simulink model "Controller"  (R2018b)
settings: configuration reference "control_config" (kept outside this file)
values from neighbouring files (symbols this model uses):
  CONTROL_EXPORT = Simulink.Parameter(CONTROL_EXPORT_VALUE)    [controller_model_init.m]
  CONTROL_PARAM = Simulink.Parameter(CONTROL_PARAM_VALUE)    [controller_model_init.m]
undefined symbols (not defined in the file or in its folder): actuator_cmd, ControlMode, DiscIntNeverNeededParam, timestamp
libraries: FMT_Model_Lib x2, simulink x1
settings Model: Creator=jc  LastModifiedBy=zouji
settings ConfigSetRef: SourceLocation=Base Workspace

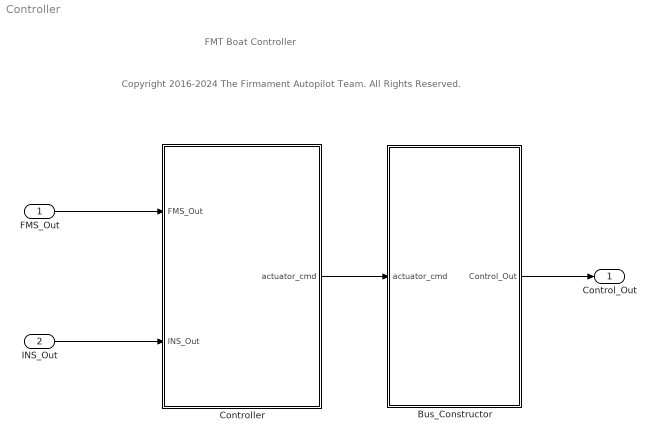
== system Controller ==
  note: FMT Boat Controller
  note: Copyright 2016-2024 The Firmament Autopilot Team. All Rights Reserved.
  FMS_Out : Inport  OutDataTypeStr=Bus: FMS_Out_Bus
  INS_Out : Inport  Port=2  OutDataTypeStr=Bus: INS_Out_Bus
  Bus_Constructor : Subsystem
  Controller : Subsystem
  Control_Out : Outport  OutDataTypeStr=Bus: Control_Out_Bus
  wires:
  Bus_Constructor/1(Control_Out) -> Control_Out/1
  INS_Out/1 -> Controller/2(INS_Out)
  FMS_Out/1 -> Controller/1(FMS_Out)
  Controller/1(actuator_cmd) -> Bus_Constructor/1(actuator_cmd)

== system Controller/Bus_Constructor ==
  actuator_cmd : Inport
  Bus Assignment : BusAssignment  AssignedSignals=actuator_cmd,timestamp
  Constant : Constant  Value=0  OutDataTypeStr=Bus: Control_Out_Bus
  timestamp : Subsystem  mask{sample_time=CONTROL_EXPORT.period}
      mask prompts: sample_time "sample time (ms)"
  Control_Out : Outport
  wires:
  actuator_cmd/1 -> Bus Assignment/2
  Constant/1 -> Bus Assignment/1
  Bus Assignment/1 -> Control_Out/1
  timestamp/1(timestamp_ms) -> Bus Assignment/3

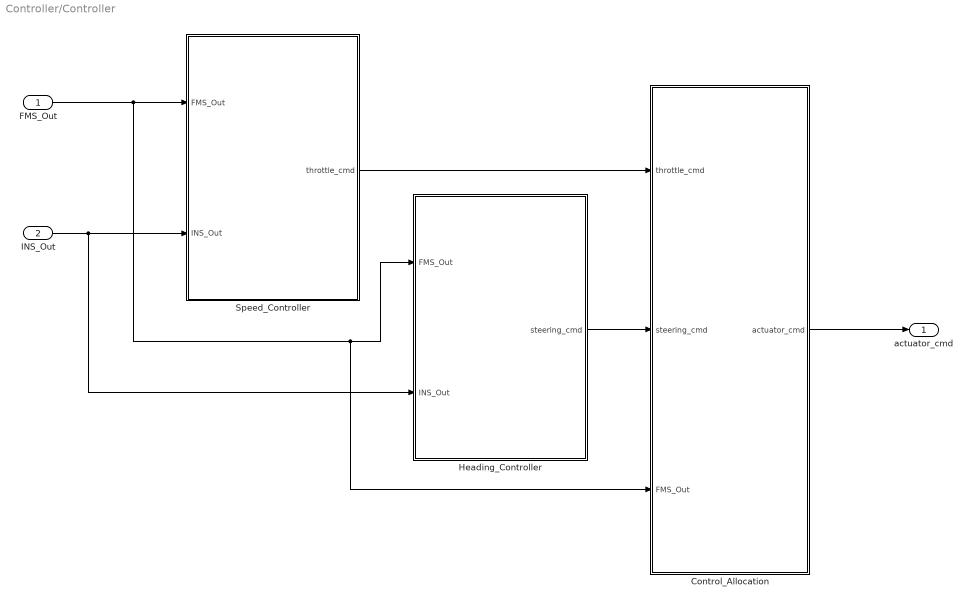
== system Controller/Controller ==
  FMS_Out : Inport
  INS_Out : Inport  Port=2
  Control_Allocation : Subsystem  Variant=on
      settings: GeneratePreprocessorConditionals=on
  Heading_Controller : Subsystem
  Speed_Controller : Subsystem
  actuator_cmd : Outport
  wires:
  FMS_Out/1 -> Control_Allocation/3(FMS_Out), Heading_Controller/1(FMS_Out), Speed_Controller/1(FMS_Out)
  INS_Out/1 -> Heading_Controller/2(INS_Out), Speed_Controller/2(INS_Out)
  Control_Allocation/1(actuator_cmd) -> actuator_cmd/1
  Speed_Controller/1(throttle_cmd) -> Control_Allocation/1(throttle_cmd)
  Heading_Controller/1(steering_cmd) -> Control_Allocation/2(steering_cmd)

== system Controller/Bus_Constructor/timestamp ==
  Constant : Constant  Value=sample_time
  Data Type Conversion : DataTypeConversion  OutDataTypeStr=uint32
  Discrete-Time Integrator : DiscreteIntegrator  IntegratorMethod=Accumulation: Forward Euler  SampleTime=-1  ICPrevOutput=DiscIntNeverNeededParam  ICPrevScaledInput=DiscIntNeverNeededParam
  timestamp_ms : Outport
  wires:
  Discrete-Time Integrator/1 -> Data Type Conversion/1
  Constant/1 -> Discrete-Time Integrator/1
  Data Type Conversion/1 -> timestamp_ms/1

== system Controller/Controller/Control_Allocation ==
  note: 1) Add Subsystem or Model blocks as valid variant choices.
      | 2) You cannot connect blocks at this level. At simulation, connectivity is automatically
      | determined, based on the active variant and port name matching.
  throttle_cmd : Inport
  steering_cmd : Inport  Port=2
  FMS_Out : Inport  Port=3
  Boat_1 : Subsystem  TreatAsAtomicUnit=on  VariantControl=AIRFRAME==1
      mask Display: image('D:\ws\FMT\FMT-Model\figures\boat_1.png');
  actuator_cmd : Outport

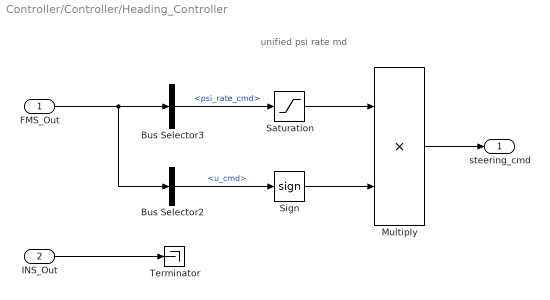
== system Controller/Controller/Heading_Controller ==
  note: unified psi rate md
  FMS_Out : Inport
  INS_Out : Inport  Port=2
  Bus Selector2 : BusSelector  OutputSignals=u_cmd
  Bus Selector3 : BusSelector  OutputSignals=psi_rate_cmd
  Multiply : Product
  Saturation : Saturate  UpperLimit=1  LowerLimit=-1
  Sign : Signum
  Terminator : Terminator
  steering_cmd : Outport
  wires:
  INS_Out/1 -> Terminator/1
  Sign/1 -> Multiply/2
  Bus Selector2/1 -> Sign/1  "<u_cmd>"
  Saturation/1 -> Multiply/1
  Multiply/1 -> steering_cmd/1
  Bus Selector3/1 -> Saturation/1  "<psi_rate_cmd>"
  FMS_Out/1 -> Bus Selector3/1, Bus Selector2/1

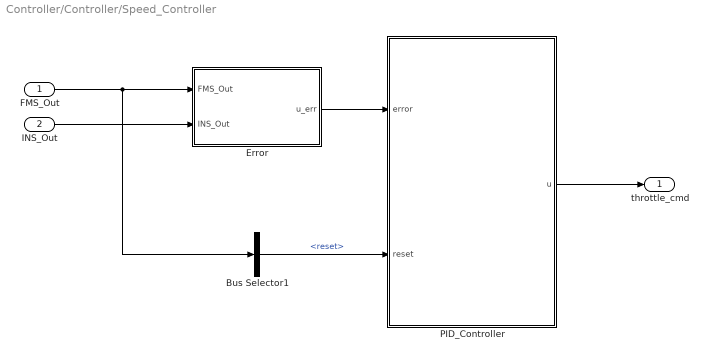
== system Controller/Controller/Speed_Controller ==
  FMS_Out : Inport
  INS_Out : Inport  Port=2
  Bus Selector1 : BusSelector  OutputSignals=reset
  Error : Subsystem
  PID_Controller : Subsystem
  throttle_cmd : Outport
  wires:
  Bus Selector1/1 -> PID_Controller/2(reset)  "<reset>"
  FMS_Out/1 -> Bus Selector1/1, Error/1(FMS_Out)
  Error/1(u_err) -> PID_Controller/1(error)
  PID_Controller/1(u) -> throttle_cmd/1
  INS_Out/1 -> Error/2(INS_Out)

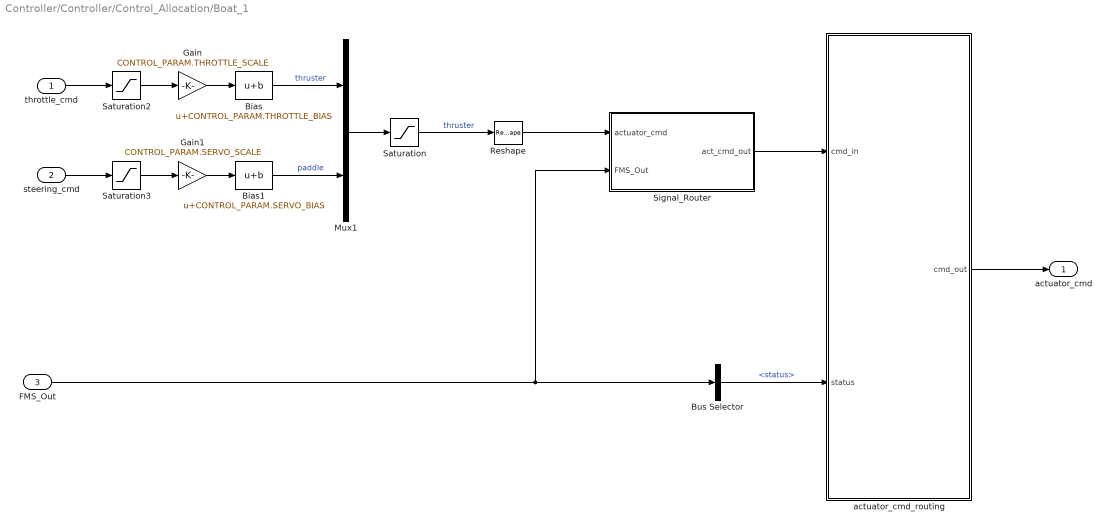
== system Controller/Controller/Control_Allocation/Boat_1 ==
  throttle_cmd : Inport
  steering_cmd : Inport  Port=2
  FMS_Out : Inport  Port=3
  Bias : Bias  Bias=CONTROL_PARAM.THROTTLE_BIAS
  Bias1 : Bias  Bias=CONTROL_PARAM.SERVO_BIAS
  Bus Selector : BusSelector  OutputSignals=status
  Gain : Gain  Gain=CONTROL_PARAM.THROTTLE_SCALE  OutDataTypeStr=uint16
  Gain1 : Gain  Gain=CONTROL_PARAM.SERVO_SCALE  OutDataTypeStr=uint16
  Mux1 : Mux  Inputs=2
  Reshape : Reshape  OutputDimensionality=Column vector (2-D)
  Saturation : Saturate  UpperLimit=2000  LowerLimit=1000
  Saturation2 : Saturate  UpperLimit=1  LowerLimit=-1
  Saturation3 : Saturate  UpperLimit=1  LowerLimit=-1
  Signal_Router : Subsystem
  actuator_cmd_routing : Subsystem
  actuator_cmd : Outport
  wires:
  Bias1/1 -> Mux1/2  "paddle"
  Gain1/1 -> Bias1/1
  Gain/1 -> Bias/1
  throttle_cmd/1 -> Saturation2/1
  steering_cmd/1 -> Saturation3/1
  Bias/1 -> Mux1/1  "thruster"
  Reshape/1 -> Signal_Router/1(actuator_cmd)
  Bus Selector/1 -> actuator_cmd_routing/2(status)  "<status>"
  Signal_Router/1(act_cmd_out) -> actuator_cmd_routing/1(cmd_in)
  FMS_Out/1 -> Signal_Router/2(FMS_Out), Bus Selector/1
  Mux1/1 -> Saturation/1
  actuator_cmd_routing/1(cmd_out) -> actuator_cmd/1
  Saturation2/1 -> Gain/1
  Saturation3/1 -> Gain1/1
  Saturation/1 -> Reshape/1  "thruster"

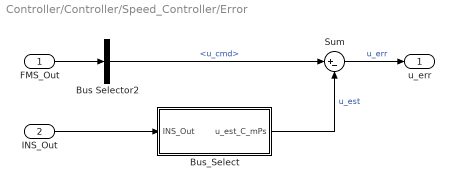
== system Controller/Controller/Speed_Controller/Error ==
  FMS_Out : Inport
  INS_Out : Inport  Port=2
  Bus Selector2 : BusSelector  OutputSignals=u_cmd
  Bus_Select : Subsystem
  Sum : Sum  Inputs=|+-
  u_err : Outport
  wires:
  FMS_Out/1 -> Bus Selector2/1
  INS_Out/1 -> Bus_Select/1(INS_Out)
  Bus_Select/1(u_est_C_mPs) -> Sum/2  "u_est"
  Bus Selector2/1 -> Sum/1  "<u_cmd>"
  Sum/1 -> u_err/1  "u_err"

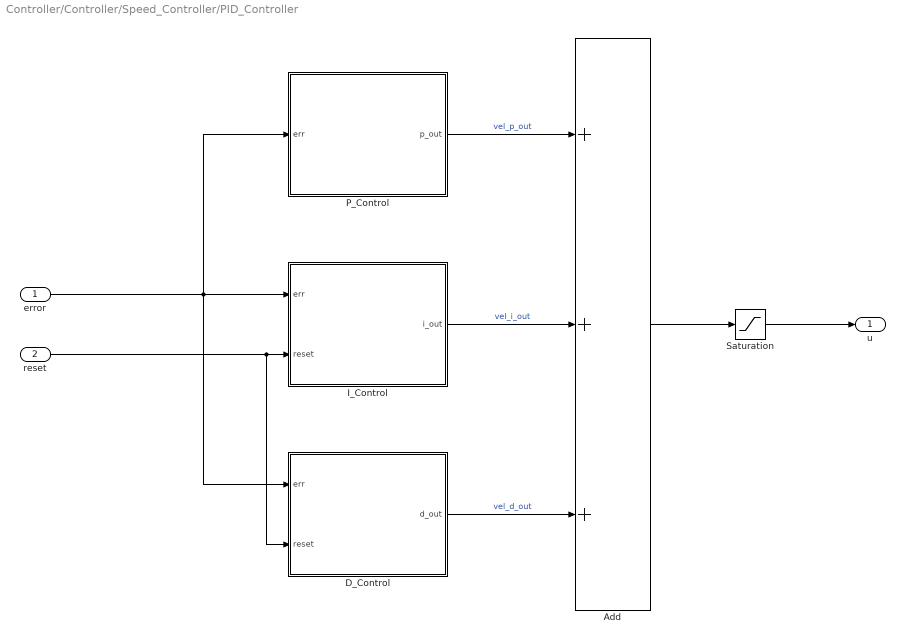
== system Controller/Controller/Speed_Controller/PID_Controller ==
  error : Inport
  reset : Inport  Port=2
  Add : Sum  Inputs=+++
  D_Control : Subsystem  mask{kd=CONTROL_PARAM.VEL_D, max_d=CONTROL_PARAM.VEL_D_MAX, min_d=CONTROL_PARAM.VEL_D_MIN}
  I_Control : Subsystem  mask{ki=CONTROL_PARAM.VEL_I, max_i=CONTROL_PARAM.VEL_I_MAX, min_i=CONTROL_PARAM.VEL_I_MIN}
  P_Control : Subsystem  mask{kp=CONTROL_PARAM.VEL_P}
  Saturation : Saturate  UpperLimit=1  LowerLimit=-1
  u : Outport
  wires:
  error/1 -> P_Control/1(err), I_Control/1(err), D_Control/1(err)
  P_Control/1(p_out) -> Add/1  "vel_p_out"
  I_Control/1(i_out) -> Add/2  "vel_i_out"
  D_Control/1(d_out) -> Add/3  "vel_d_out"
  reset/1 -> I_Control/2(reset), D_Control/2(reset)
  Add/1 -> Saturation/1
  Saturation/1 -> u/1

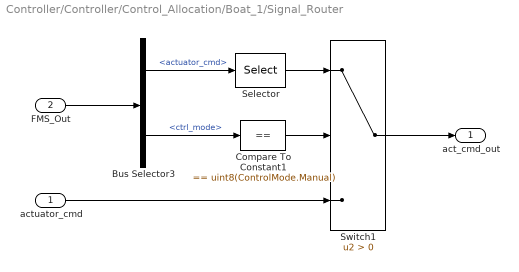
== system Controller/Controller/Control_Allocation/Boat_1/Signal_Router ==
  actuator_cmd : Inport
  FMS_Out : Inport  Port=2
  Bus Selector3 : BusSelector  OutputSignals=actuator_cmd,ctrl_mode
  Compare To Constant1 : simulink/Logic and Bit Operations/Compare To Constant  relop===  const=uint8(ControlMode.Manual)  OutDataTypeStr=boolean
  Selector : Selector  InputPortWidth=16  IndexOptions=Index vector (dialog)  Indices=[1 2]  OutputSizes=1
  Switch1 : Switch  Criteria=u2 > Threshold
  act_cmd_out : Outport
  wires:
  Compare To Constant1/1 -> Switch1/2
  Bus Selector3/1 -> Selector/1  "<actuator_cmd>"
  Bus Selector3/2 -> Compare To Constant1/1  "<ctrl_mode>"
  actuator_cmd/1 -> Switch1/3
  FMS_Out/1 -> Bus Selector3/1
  Switch1/1 -> act_cmd_out/1
  Selector/1 -> Switch1/1

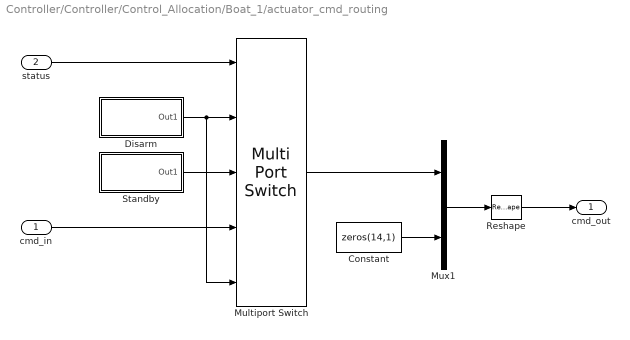
== system Controller/Controller/Control_Allocation/Boat_1/actuator_cmd_routing ==
  cmd_in : Inport
  status : Inport  Port=2
  Constant : Constant  Value=zeros(14,1)  VectorParams1D=off  OutDataTypeStr=uint16
  Disarm : Subsystem
  Multiport Switch : MultiPortSwitch  DataPortForDefault=Additional data port  DiagnosticForDefault=None
  Mux1 : Mux  Inputs=2
  Reshape : Reshape  OutputDimensionality=Customize  OutputDimensions=[16,1]
  Standby : Subsystem
  cmd_out : Outport
  wires:
  Reshape/1 -> cmd_out/1
  Constant/1 -> Mux1/2
  Mux1/1 -> Reshape/1
  status/1 -> Multiport Switch/1
  Multiport Switch/1 -> Mux1/1
  cmd_in/1 -> Multiport Switch/4
  Disarm/1(Out1) -> Multiport Switch/5, Multiport Switch/2
  Standby/1(Out1) -> Multiport Switch/3

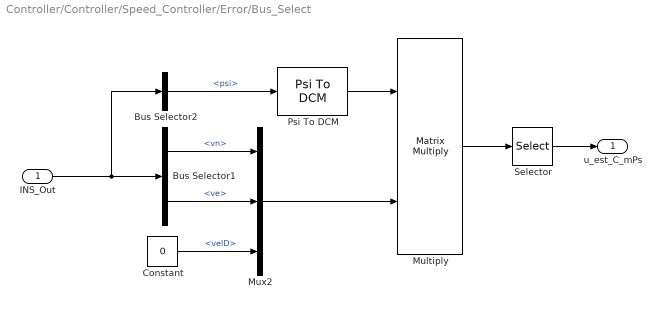
== system Controller/Controller/Speed_Controller/Error/Bus_Select ==
  INS_Out : Inport
  Bus Selector1 : BusSelector  OutputSignals=vn,ve
  Bus Selector2 : BusSelector  OutputSignals=psi
  Constant : Constant  Value=0  OutDataTypeStr=single
  Multiply : Product  Multiplication=Matrix(*)
  Mux2 : Mux  Inputs=3
  Psi To DCM : FMT_Model_Lib/Transformation/Psi To DCM
      settings: SourceProductName=FMT Toolbox
  Selector : Selector  InputPortWidth=3  IndexOptions=Index vector (dialog)  Indices=1  OutputSizes=1
  u_est_C_mPs : Outport
  wires:
  Psi To DCM/1 -> Multiply/1
  Bus Selector2/1 -> Psi To DCM/1  "<psi>"
  Constant/1 -> Mux2/3  "<velD>"
  Mux2/1 -> Multiply/2
  Bus Selector1/2 -> Mux2/2  "<ve>"
  Bus Selector1/1 -> Mux2/1  "<vn>"
  INS_Out/1 -> Bus Selector2/1, Bus Selector1/1
  Multiply/1 -> Selector/1
  Selector/1 -> u_est_C_mPs/1

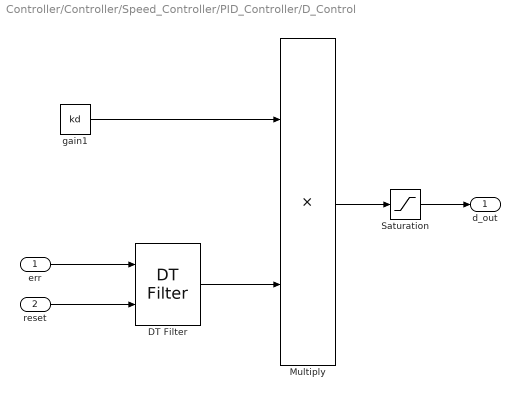
== system Controller/Controller/Speed_Controller/PID_Controller/D_Control ==
  err : Inport
  reset : Inport  Port=2
  DT Filter : FMT_Model_Lib/Filter/DT Filter  fc=30
      settings: SourceProductName=FMT Toolbox
  Multiply : Product  OutDataTypeStr=Inherit: Same as first input
  Saturation : Saturate  UpperLimit=max_d  LowerLimit=min_d
  gain1 : Constant  Value=kd  OutDataTypeStr=single
  d_out : Outport
  wires:
  err/1 -> DT Filter/1
  Multiply/1 -> Saturation/1
  Saturation/1 -> d_out/1
  reset/1 -> DT Filter/2
  gain1/1 -> Multiply/1
  DT Filter/1 -> Multiply/2

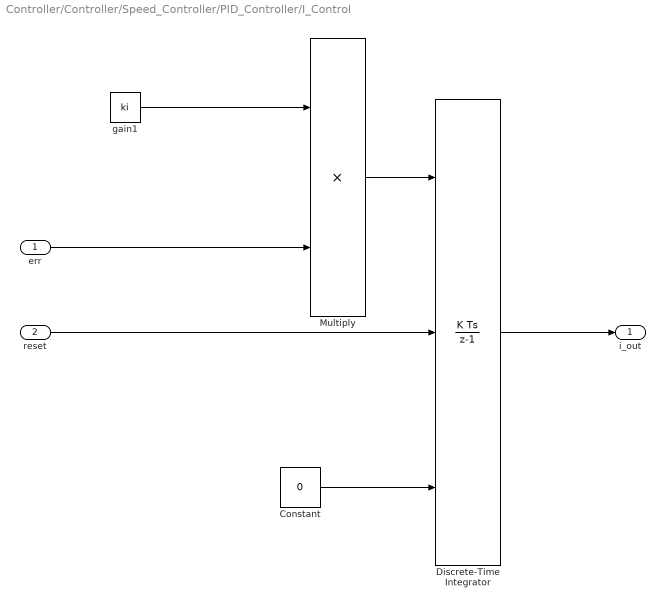
== system Controller/Controller/Speed_Controller/PID_Controller/I_Control ==
  err : Inport
  reset : Inport  Port=2
  Constant : Constant  Value=0  OutDataTypeStr=single
  Discrete-Time Integrator : DiscreteIntegrator  ExternalReset=level  InitialConditionSource=external  SampleTime=-1  LimitOutput=on  UpperSaturationLimit=max_i  LowerSaturationLimit=min_i  ICPrevOutput=DiscIntNeverNeededParam  ICPrevScaledInput=DiscIntNeverNeededParam
  Multiply : Product  OutDataTypeStr=Inherit: Same as first input
  gain1 : Constant  Value=ki  OutDataTypeStr=single
  i_out : Outport
  wires:
  err/1 -> Multiply/2
  reset/1 -> Discrete-Time Integrator/2
  Constant/1 -> Discrete-Time Integrator/3
  Discrete-Time Integrator/1 -> i_out/1
  gain1/1 -> Multiply/1
  Multiply/1 -> Discrete-Time Integrator/1

== system Controller/Controller/Speed_Controller/PID_Controller/P_Control ==
  err : Inport
  Multiply : Product  OutDataTypeStr=Inherit: Same as first input
  gain1 : Constant  Value=kp  OutDataTypeStr=single
  p_out : Outport
  wires:
  err/1 -> Multiply/2
  Multiply/1 -> p_out/1
  gain1/1 -> Multiply/1

== system Controller/Controller/Control_Allocation/Boat_1/actuator_cmd_routing/Disarm ==
  Disarm : Constant  Value=CONTROL_PARAM.THROTTLE_BIAS  VectorParams1D=off  OutDataTypeStr=uint16
  Mux : Mux  Inputs=2
  Out1 : Outport
  wires:
  Mux/1 -> Out1/1
  Disarm/1 -> Mux/2, Mux/1

== system Controller/Controller/Control_Allocation/Boat_1/actuator_cmd_routing/Standby ==
  Mux : Mux  Inputs=2
  Standby : Constant  Value=CONTROL_PARAM.SERVO_BIAS  VectorParams1D=off  OutDataTypeStr=uint16
  Out1 : Outport
  wires:
  Standby/1 -> Mux/2, Mux/1
  Mux/1 -> Out1/1
